simulink model "ParallelClientExample"  (R2018a)
settings: Solver=VariableStepAuto  StartTime=0.0  StopTime=30  RelTol=1e-3
StartFcn:
  | StartUDPModelSim({'ParallelServer1Example','ParallelServer2Example'})
StopFcn:
  | delete(gcp('nocreate'))
libraries: transmit_lib x4
settings Model: Creator=hfeng  LastModifiedBy=grouleau
settings OptimizationCC: EnhancedBackFolding=on  OptimizeBlockOrder=speed  DifferentSizesBufferReuse=on  OptimizationCustomize=off

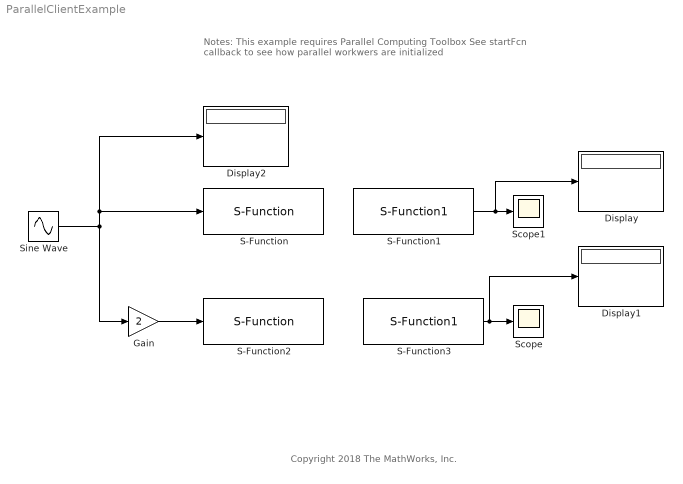
== system ParallelClientExample ==
  note: Copyright 2018 The MathWorks, Inc.
  note: Notes:
      | This example requires Parallel Computing Toolbox
      | See startFcn callback to see how parallel workwers are initialized
  Display : Display
  Display1 : Display
  Display2 : Display
  Gain : Gain  Gain=2
  S-Function : transmit_lib/S-Function  Priority=1  hostname=localhost  portnumber=8099  datawidth=3  stepsize=0.1
      settings: SourceProductName=The database C:\Users\grouleau\AppData\Roaming\MathWorks\MATLAB\R2018a\slblocks_master.db is locked, or a table in the database is locked. (database is locked)
      settings: AttributesFormatString=|
      | %<hostname>
      | %<portnumber>
      | Priority: %<Priority>
  S-Function1 : transmit_lib/S-Function1  Priority=3  hostname=localhost  portnumber=8090  datawidth=3  stepsize=0.1
      settings: SourceProductName=The database C:\Users\grouleau\AppData\Roaming\MathWorks\MATLAB\R2018a\slblocks_master.db is locked, or a table in the database is locked. (database is locked)
      settings: AttributesFormatString=|
      | %<hostname>
      | %<portnumber>
      | Priority: %<Priority>
  S-Function2 : transmit_lib/S-Function  Priority=2  hostname=localhost  portnumber=8092  datawidth=3  stepsize=0.1
      settings: SourceProductName=The database C:\Users\grouleau\AppData\Roaming\MathWorks\MATLAB\R2018a\slblocks_master.db is locked, or a table in the database is locked. (database is locked)
      settings: AttributesFormatString=|
      | %<hostname>
      | %<portnumber>
      | Priority: %<Priority>
  S-Function3 : transmit_lib/S-Function1  Priority=4  hostname=localhost  portnumber=8093  datawidth=3  stepsize=0.1
      settings: SourceProductName=The database C:\Users\grouleau\AppData\Roaming\MathWorks\MATLAB\R2018a\slblocks_master.db is locked, or a table in the database is locked. (database is locked)
      settings: AttributesFormatString=|
      | %<hostname>
      | %<portnumber>
      | Priority: %<Priority>
  Scope : Scope
  Scope1 : Scope
  Sine Wave : Sin  SineType=Sample based  Amplitude=rand(3,1)  Samples=11  SampleTime=0.1
  wires:
  Sine Wave/1 -> Display2/1, S-Function/1, Gain/1
  S-Function3/1 -> Display1/1, Scope/1
  S-Function1/1 -> Display/1, Scope1/1
  Gain/1 -> S-Function2/1
